simulink model "exp03p02"  (R2021a)
settings: Solver=VariableStepAuto  StartTime=0.0  StopTime=10.0  RelTol=1e-3
libraries: spsThyristorLib x4, spsSeriesRLCBranchLib x3, spsVoltageMeasurementLib x2, spsACVoltageSourceLib x1, spsIGBTDiodeLib x1, spsMeanLib x1, spsPLLLib x1, spsSampleandHoldLib x1, spspowerguiLib x1
settings Model: Creator=User  LastModifiedBy=User

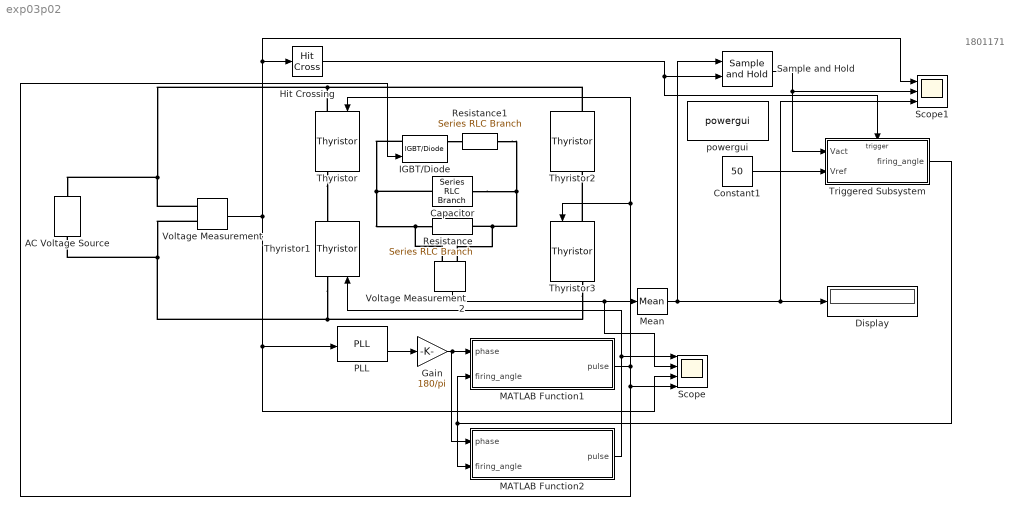
== system exp03p02 ==
  note: 1801171
  AC Voltage Source : spsACVoltageSourceLib/AC Voltage Source  Amplitude=100  Phase=0  Frequency=50  SampleTime=0  Measurements=None  BusType=swing  Pref=10e3  Qref=0  Qmin=-inf  Qmax=+inf
  Capacitor : spsSeriesRLCBranchLib/Series RLC Branch  LConnTagsString=__new0  RConnTagsString=__new0  BranchType=C  Resistance=1000  Inductance=1e-3  SetiL0=off  InitialCurrent=0  Capacitance=1e-6  Setx0=off  InitialVoltage=0  Measurements=None
  Constant1 : Constant  Value=50  SampleTime=0.0001
  Display : Display
  Gain : Gain  Gain=180/pi
  Hit Crossing : HitCross
  IGBT/Diode : spsIGBTDiodeLib/IGBT//Diode  Ron=1e-3  Rs=1e5  Cs=inf  Measurements=on
  MATLAB Function1 : MATLAB Function  TreatAsAtomicUnit=on
  MATLAB Function2 : MATLAB Function  TreatAsAtomicUnit=on
  Mean : spsMeanLib/Mean  Freq=50  Vinit=0  Ts=0
  PLL : spsPLLLib/PLL  Fmin=45  Par_Init=[0, 50]  ParK=[180, 3200, 1]  TcD=1e-4  MaxRateChangeFreq=12  FilterCutOffFreq=25  Ts=0.0001  AGC=on
      settings: SourceProductBaseCode=PS
  Resistance : spsSeriesRLCBranchLib/Series RLC Branch  LConnTagsString=__new0  RConnTagsString=__new0  BranchType=R  Resistance=1000  Inductance=1e-3  SetiL0=off  InitialCurrent=0  Capacitance=1e-6  Setx0=off  InitialVoltage=0  Measurements=None
  Resistance1 : spsSeriesRLCBranchLib/Series RLC Branch  LConnTagsString=__new0  RConnTagsString=__new0  BranchType=R  Resistance=1000  Inductance=1e-3  SetiL0=off  InitialCurrent=0  Capacitance=1e-6  Setx0=off  InitialVoltage=0  Measurements=None
  Sample and Hold : spsSampleandHoldLib/Sample and Hold  ic=0  Ts=0
      settings: SourceProductBaseCode=PS
  Scope : Scope  NumInputPorts=4
  Scope1 : Scope  NumInputPorts=3
  Thyristor{,1..3} (4 alike) : spsThyristorLib/Thyristor  Ron=0.001  Lon=0  Vf=0.8  IC=0  Rs=500  Cs=250e-9  Measurements=on
  Triggered Subsystem : Subsystem  TreatAsAtomicUnit=on
  Voltage Measurement : spsVoltageMeasurementLib/Voltage Measurement  PhasorSimulation=off  OutputType=Complex  PSBequivalent=0
  Voltage Measurement2 : spsVoltageMeasurementLib/Voltage Measurement  PhasorSimulation=off  OutputType=Complex  PSBequivalent=0
  powergui : spspowerguiLib/powergui  Priority=1  SimulationMode=Discrete  SampleTime=50e-6  frequency=60  Iterations=50  frequencyindice=0  Pbase=100e6  ErrMax=1e-4  UnitsV=kV  UnitsW=MW  buscounter=0  FunctionMessages=off  echomessages=off  EnableUseOfTLC=off  CurrentSourceSwitches=off  DisableSnubberDevices=off  DisableRonSwitches=off  DisableVfSwitches=off  DisplayEquations=off  AutomaticDiscreteSolvers=off  SolverType=Tustin/Backward Euler (TBE)  Interpol=off  ExternalGateDelay=off  methode=off  Ts=100  x0status=blocks  SPID=on  SwTol=0  HookPort=off  NonlinearTolerance=1e-4  nMaxIteration=100  ContinueOnMaxIteration=off  RestoreLinks=warning  ResistiveCurrentMeasurement=off  Frange=[0:2:500]  Ylog=off  Xlog=on  ShowGrid=off  save=off  variable=ZData  structure=0  ZoomFFT=off  StartTime=0.0  cycles=1  DisplayStyle=1  fundamental=60  FreqAxis=off  MaxFrequency=1000  frequencyindicesteady=1  RmsSteady=1  display=off
  wires:
  Voltage Measurement/1 -> Hit Crossing/1, Scope1/1, PLL/1, Scope/3
  Mean/1 -> Display/1, Scope1/3, Sample and Hold/1
  PLL/2 -> Gain/1
  Triggered Subsystem/1(firing_angle) -> MATLAB Function1/2(firing_angle), MATLAB Function2/2(firing_angle)
  Gain/1 -> MATLAB Function1/1(phase), MATLAB Function2/1(phase)
  Hit Crossing/1 -> Sample and Hold/2, Triggered Subsystem/Trigger
  Sample and Hold/1 -> Triggered Subsystem/1(Vact), Scope1/2
  Constant1/1 -> Triggered Subsystem/2(Vref)
  MATLAB Function1/1(pulse) -> Thyristor3/1, Thyristor/1, IGBT/Diode/1, Scope/4
  Voltage Measurement2/1 -> Scope/2, Mean/1
  MATLAB Function2/1(pulse) -> Thyristor1/1, Scope/1
  connections:
  Thyristor/LConn1 -- Voltage Measurement/LConn1 -- AC Voltage Source/RConn1 -- Thyristor2/RConn1
  Voltage Measurement/LConn2 -- Thyristor1/LConn1 -- Thyristor3/RConn1 -- AC Voltage Source/LConn1
  IGBT/Diode/RConn1 -- Resistance1/LConn1
  Thyristor/RConn1 -- Thyristor1/RConn1
  IGBT/Diode/LConn1 -- Voltage Measurement2/LConn1 -- Resistance/RConn1 -- Capacitor/LConn1
  Resistance1/RConn1 -- Voltage Measurement2/LConn2 -- Resistance/LConn1 -- Capacitor/RConn1
  Thyristor3/LConn1 -- Thyristor2/LConn1

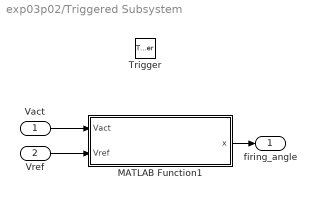
== system exp03p02/Triggered Subsystem ==
  Vact : Inport
  Vref : Inport  Port=2
  Trigger : TriggerPort  VariantControl=(inherit)
  MATLAB Function1 : MATLAB Function  TreatAsAtomicUnit=on
  firing_angle : Outport
  wires:
  Vact/1 -> MATLAB Function1/1(Vact)
  Vref/1 -> MATLAB Function1/2(Vref)
  MATLAB Function1/1(x) -> firing_angle/1

== matlab function exp03p02/Triggered Subsystem/MATLAB Function1 ==
  data: Vact input; x output; Vref input
function x = fcn(Vact,Vref)
%codegen
persistent firing_angle
if isempty(firing_angle),firing_angle=10,end;
step = 0.5;
if Vact<Vref
    firing_angle = firing_angle-step;
    if firing_angle<0
        firing_angle = 0;
    end
elseif Vact>Vref
    firing_angle = firing_angle+step;
    if firing_angle>180
        firing_angle = 180;
    else
        firing_angle = firing_angle;
    end
end
x = firing_angle;
end

== matlab function exp03p02/MATLAB Function2 ==
  data: phase input; pulse output; firing_angle input
function pulse = negative(phase,firing_angle)
%codegen
pulse_width = 10;
if (phase>=(firing_angle+180))&&(phase<=min((firing_angle+pulse_width+180),360))
    pulse = 1;
else
    pulse = 0;
end
end

== matlab function exp03p02/MATLAB Function1 ==
  data: phase input; pulse output; firing_angle input
function pulse = positive(phase,firing_angle)
%codegen
pulse_width = 10;
if (phase>=firing_angle)&&(phase<=min((firing_angle+pulse_width),180))
    pulse = 1;
else
    pulse = 0;
end
end
